simulink model "Driver_Glider"  (R2020b)
settings: Solver=ode45  StartTime=0.0  StopTime=TimeUS06  MaxStep=.1  RelTol=1e-3  EnableMultiTasking=on
PostLoadFcn:
  | GliderDir = pwd;
  | 
  | cd ..\;
  | SimulinkDir = pwd;
  | addpath(SimulinkDir);
  | 
  | cd(GliderDir);
model workspace (MAT data in the model file):
  DrCycles.C505 = [0 1 2 3 4 5 6 7 8 9 10 11 ... (1012 elements, 506x2)]
  DrCycles.FTP = [0 1 2 3 4 5 6 7 8 9 10 11 ... (4956 elements, 2478x2)]
  DrCycles.UDDS = [0 1 2 3 4 5 6 7 8 9 10 11 ... (2746 elements, 1373x2)]
  DrCycles.HWFET = [0 1 2 3 4 5 6 7 8 9 10 11 ... (1532 elements, 766x2)]
  DrCycles.US06 = [0 1 2 3 4 5 6 7 8 9 10 11 ... (1194 elements, 597x2)]
  DrCycles.US06City = [0 1 2 3 4 5 6 7 8 9 10 11 ... (466 elements, 233x2)]
  DrCycles.US06Hwy = [0 1 2 3 4 5 6 7 8 9 10 11 ... (742 elements, 371x2)]
  DriverPic = [255 255 255 255 255 255 255 255 255 255 255 255 ... (1049040 elements, 940x372x3)]
  TimeHWFET = 765
  TimeUDDS = 1372
  TimeUS06 = 596
  VehiclePic = [252 252 252 252 252 252 252 252 252 252 252 252 ... (1047540 elements, 316x1105x3)]
  aeroDragCoeff = 0.38
  airDensity = 1.23
  frontArea = 2.1
  gravity = 9.81
  inclinationAngle = 0
  inertialMassVeh = 2392
  massVeh = 2300
  rollingResistCoeff = 0.01
libraries: mpclib x1, pid_lib x1, Driver_Glider_Library x1
(part 1 of 2)
CloseFcn:
  | rmpath(SimulinkDir);
  | clear GliderDir SimulinkDir;
settings Model: Creator=EduardoMarquez  LastModifiedBy=Lenovo
settings DataIOCC: ExternalInput=[US06]  LimitDataPoints=on  SaveFormat=Array  SignalLoggingSaveFormat=ModelDataLogs  ReturnWorkspaceOutputs=off
settings OptimizationCC: LifeSpan=inf
settings DebuggingCC: SolverPrmCheckMsg=warning  SFUnexpectedBacktrackingDiag=warning  SFNoUnconditionalDefaultTransitionDiag=warning  SFExecutionAtInitializationDiag=none  ArithmeticOperatorsInVariantConditions=warning
settings HardwareCC: ProdBitPerPointer=32  ProdBitPerSizeT=32  ProdBitPerPtrDiffT=32  ProdLargestAtomicFloat=None  ProdIntDivRoundTo=Undefined  ProdEndianess=Unspecified  ProdWordSize=32  ProdHWDeviceType=32-bit Generic
settings ModelReferenceCC: PropagateSignalLabelsOutOfModel=off
settings SFSimCC: SimUseLocalCustomCode=off  CustomCodeUndefinedFunction=UseInterfaceOnly
settings RTWCC: RTWUseLocalCustomCode=off
settings CodeAppCC: StateflowObjectComments=on
settings GRTTargetCC: TargetLangStandard=C89/C90 (ANSI)
settings ConfigComp: CovMetricSettings=dw  CovSaveCumulativeToWorkspaceVar=on  CovSaveSingleToWorkspaceVar=on  CovExternalEMLEnable=off  CovSFcnEnable=off

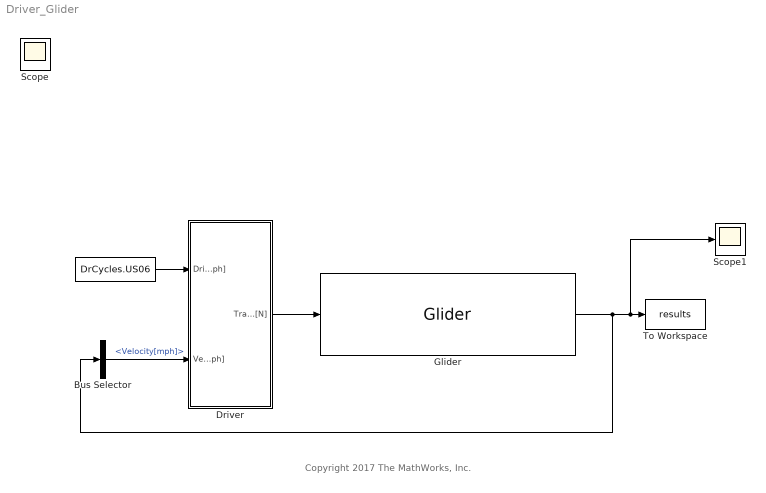
== system Driver_Glider ==
  note: Copyright 2017 The MathWorks, Inc.
  " " : FromWorkspace  Tag=DriveCycle  VariableName=DrCycles.US06
  Bus Selector : BusSelector  OutputSignals=Velocity[mph]
  Driver : Subsystem
      mask Display: image('C:\Users\Lenovo\OneDrive\Documents\vehicle-modeling-master\vehicle-modeling-master\VehicleModeling4p0\1_Simulink\DriverPic.jpg'); % Use "Edit Image" on toolstrip to change.
  Glider : Driver_Glider_Library/Glider  SystemSampleTime=-1  VariantActivationTime=update diagram  Latency=0  AutoFrameSizeCalculation=off
      mask Display: image('C:\Users\Lenovo\OneDrive\Documents\vehicle-modeling-master\vehicle-modeling-master\VehicleModeling4p0\1_Simulink\VehiclePic.jpg'); % Use "Edit Image" on toolstrip to change.
  Scope1 : Scope
  To Workspace : ToWorkspace  VariableName=results  SaveFormat=Timeseries  SampleTime=-1
  Scope : Scope
  wires:
  " "/1 -> Driver/1(DriveCycleSpeed[mph])
  Driver/1(TractiveForce[N]) -> Glider/1
  Glider/1 -> Scope1/1, To Workspace/1, Bus Selector/1
  Bus Selector/1 -> Driver/2(VehicleSpeed[mph])  "<Velocity[mph]>"
